simulink model "Q2b"  (R2023b)
settings: Solver=FixedStepAuto  StartTime=0.0  StopTime=90  FixedStep=0.01  RelTol=1e-3
undefined symbols (not defined in the file or in its folder): Continuous, Time
libraries: ctrlSharedLib x1
settings Model: Creator=Ali  LastModifiedBy=Ali

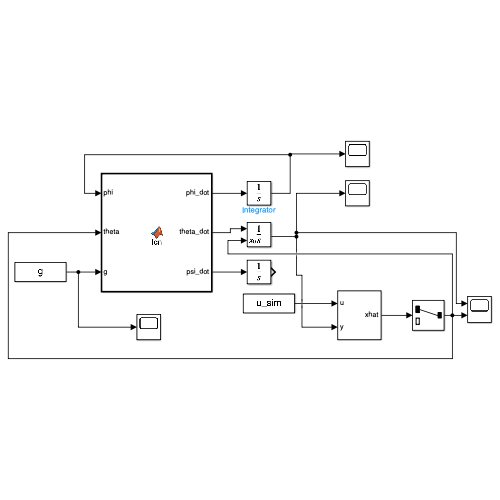
[thumbnail: Simulink's stored preview of the top-level diagram]
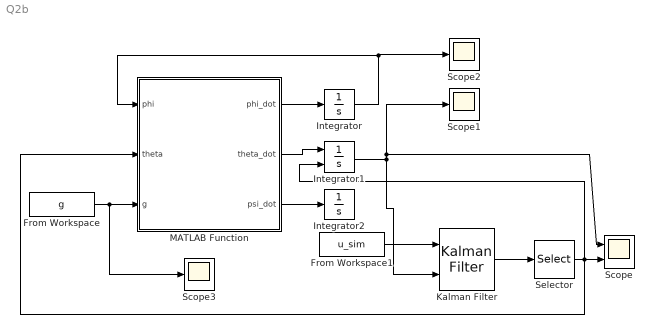
== system Q2b ==
  From Workspace : FromWorkspace  VariableName=g
  From Workspace1 : FromWorkspace  VariableName=u_sim
  Integrator : Integrator
  Integrator1 : Integrator  InitialConditionSource=external
  Integrator2 : Integrator
  Kalman Filter : ctrlSharedLib/Kalman Filter  TimeDomain=Continuous-Time  UseCurrentEstimator=on  ModelSource=Individual A, B, C, D matrices  ModelSourceVariable=ss(0.95,1,1,0,1)  A=[0 1; 0 0]  B=[0; 0.72]  C=[1, 0]  D=0  NumberOfStates=1  NumberOfInputs=1  NumberOfOutputs=1  InitialEstimateSource=Dialog  X0=0  P0=10  UseK=off  UseGH=off  NumberOfProcessNoiseInputs=1  G=1  TimeInvariantG=on  H=0  TimeInvariantH=on  Q=0.5  TimeInvariantQ=on  R=1  TimeInvariantR=on  N=0  TimeInvariantN=on  AddInputPort=on  AddEnablePort=off  OutputEstimatedY=off  OutputP=off  Ts=-1
  MATLAB Function : MATLAB Function  TreatAsAtomicUnit=on
  Scope : Scope  NumInputPorts=2
  Scope1 : Scope
  Scope2 : Scope
  Scope3 : Scope
  Selector : Selector  InputPortWidth=2  IndexOptions=Index vector (dialog)  Indices=[1]  OutputSizes=1
  wires:
  From Workspace1/1 -> Kalman Filter/1
  Kalman Filter/1 -> Selector/1
  Selector/1 -> Integrator1/2, MATLAB Function/2(theta), Scope/2
  MATLAB Function/1(phi_dot) -> Integrator/1
  MATLAB Function/2(theta_dot) -> Integrator1/1
  MATLAB Function/3(psi_dot) -> Integrator2/1
  Integrator/1 -> Scope2/1, MATLAB Function/1(phi)
  Integrator1/1 -> Scope/1, Scope1/1, Kalman Filter/2
  From Workspace/1 -> Scope3/1, MATLAB Function/3(g)

== matlab function Q2b/MATLAB Function ==
  data: phi input; phi_dot output; theta input; g input; theta_dot output; psi_dot output
function [phi_dot, theta_dot, psi_dot] = fcn(phi, theta, g)
p = g(1);
q = g(1);
r = g(1);
phi_dot = p + tan(theta)*(q*sin(phi) + r*cos(phi))*tan(theta);
theta_dot = q*cos(phi) - r*sin(phi);
psi_dot = (q*sin(phi) + r*cos(phi))/cos(theta);
